simulink model "magPhase"  (R2024a)
settings: Solver=FixedStepDiscrete  StartTime=0.0  StopTime=1  RelTol=1e-3
undefined symbols (not defined in the file): dx, dy
libraries: visionsinks x4, visionsources x1
Description:
  | Sobel Edge Detection Using the MATLAB(R) Function Block
  | This example shows how to use HDL Coder(TM) to check,
  | generate, and verify HDL code for a Sobel Edge Detection
  | block built using the MATLAB Function block.
settings Model: FPTRunName=Active  Creator=The MathWorks, Inc.  LastModifiedBy=dskap
settings SolverCC: AlgebraicLoopSolver=TrustRegion
settings DataIOCC: LimitDataPoints=on  SaveFormat=Array  SignalLogging=off  ReturnWorkspaceOutputs=off
settings OptimizationCC: BlockReduction=off  ConditionallyExecuteInputs=off  DefaultParameterBehavior=Inlined  ExpressionDepthLimit=2147483647  InitFltsAndDblsToZero=on  EfficientMapNaN2IntZero=off  LifeSpan=inf
settings DebuggingCC: AlgebraicLoopMsg=error  SaveWithParameterizedLinksMsg=none  UnderspecifiedInitializationDetection=Classic  MergeDetectMultiDrivingBlocksExec=none  SignalResolutionControl=TryResolveAllWithWarning  MultiTaskDSMMsg=warning  MultiTaskCondExecSysMsg=none  SingleTaskRateTransMsg=error  IntegerOverflowMsg=none  ParameterPrecisionLossMsg=none  FcnCallInpInsideContextMsg=warning  UnconnectedInputMsg=warning  UnconnectedOutputMsg=warning  UnconnectedLineMsg=warning  AllowSymbolicDim=off  StateNameClashWarn=warning  StrictBusMsg=ErrorOnBusTreatedAsVector  SFUnexpectedBacktrackingDiag=warning  SFNoUnconditionalDefaultTransitionDiag=warning  SFExecutionAtInitializationDiag=none  IntegerSaturationMsg=none  ArithmeticOperatorsInVariantConditions=warning
settings HardwareCC: ProdBitPerPointer=32  ProdBitPerSizeT=32  ProdBitPerPtrDiffT=32  ProdLargestAtomicFloat=None  ProdIntDivRoundTo=Undefined  ProdEndianess=Unspecified  ProdWordSize=32  ProdHWDeviceType=ASIC/FPGA  TargetHWDeviceType=32-bit Generic  ProdEqTarget=off
settings ModelReferenceCC: EnableRefExpFcnMdlSchedulingChecks=on  PropagateSignalLabelsOutOfModel=off
settings SFSimCC: SimUseLocalCustomCode=off  CustomCodeUndefinedFunction=UseInterfaceOnly
settings RTWCC: RTWUseLocalCustomCode=off  GPUComputeCapability=3.5  DLArmComputeVersion=19.05
settings CodeAppCC: StateflowObjectComments=on
settings GRTTargetCC: TargetFcnLib=ansi_tfl_tmw.mat  TargetLangStandard=C89/C90 (ANSI)  CombineOutputUpdateFcns=off  GRTInterface=on
settings ConfigComp: CovMetricSettings=dw  CovSaveCumulativeToWorkspaceVar=on  CovSaveSingleToWorkspaceVar=on  CovExternalEMLEnable=off

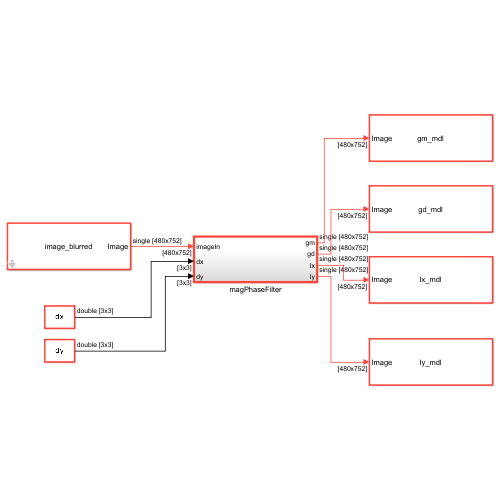
[thumbnail: Simulink's stored preview of the top-level diagram]
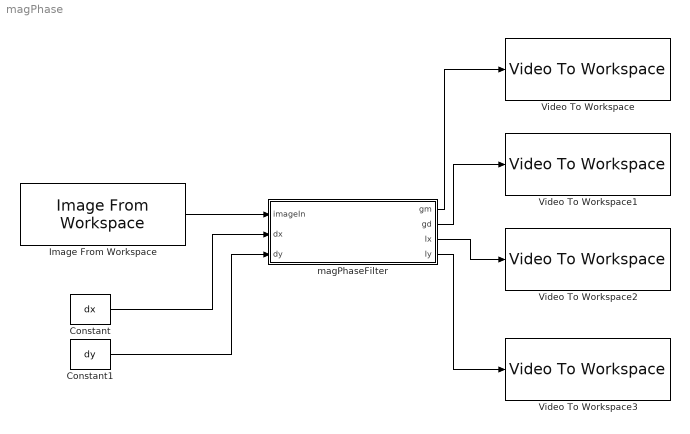
== system magPhase ==
  Constant : Constant  Value=dx  SampleTime=-1
  Constant1 : Constant  Value=dy  SampleTime=-1
  Image From Workspace : visionsources/Image From Workspace  Tag=vipblks_nd  ImageValue=image_blurred  Ts=1  imagePorts=One multidimensional signal  OutPortLabels=R|G|B  ImageDataType=Inherit from 'Value'  Signed=on  WordLength=16  sdImageDataType=sfix(16)  FractionLengthMode=User-defined  FractionLength=15
  Video To Workspace : visionsinks/Video To Workspace  VariableName=gm_mdl  NumInputs=1  DataLimit=1  DecimationFactor=1  LogFi=off  InPortLabels=R|G|B
  Video To Workspace1 : visionsinks/Video To Workspace  VariableName=gd_mdl  NumInputs=1  DataLimit=1  DecimationFactor=1  LogFi=off  InPortLabels=R|G|B
  Video To Workspace2 : visionsinks/Video To Workspace  VariableName=Ix_mdl  NumInputs=1  DataLimit=1  DecimationFactor=1  LogFi=off  InPortLabels=R|G|B
  Video To Workspace3 : visionsinks/Video To Workspace  VariableName=Iy_mdl  NumInputs=1  DataLimit=1  DecimationFactor=1  LogFi=off  InPortLabels=R|G|B
  magPhaseFilter : Subsystem  TreatAsAtomicUnit=on
  wires:
  Image From Workspace/1 -> magPhaseFilter/1(imageIn)
  magPhaseFilter/1(gm) -> Video To Workspace/1
  magPhaseFilter/2(gd) -> Video To Workspace1/1
  Constant/1 -> magPhaseFilter/2(dx)
  Constant1/1 -> magPhaseFilter/3(dy)
  magPhaseFilter/3(Ix) -> Video To Workspace2/1
  magPhaseFilter/4(Iy) -> Video To Workspace3/1

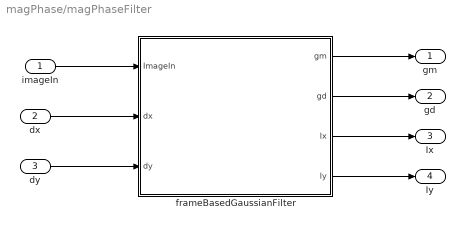
== system magPhase/magPhaseFilter ==
  imageIn : Inport
  dx : Inport  Port=2
  dy : Inport  Port=3
  frameBasedGaussianFilter : MATLAB Function  TreatAsAtomicUnit=on
  gm : Outport
  gd : Outport  Port=2
  Ix : Outport  Port=3
  Iy : Outport  Port=4
  wires:
  imageIn/1 -> frameBasedGaussianFilter/1(ImageIn)
  frameBasedGaussianFilter/1(gm) -> gm/1
  dx/1 -> frameBasedGaussianFilter/2(dx)
  dy/1 -> frameBasedGaussianFilter/3(dy)
  frameBasedGaussianFilter/2(gd) -> gd/1
  frameBasedGaussianFilter/3(Ix) -> Ix/1
  frameBasedGaussianFilter/4(Iy) -> Iy/1

== matlab function magPhase/magPhaseFilter/frameBasedGaussianFilter ==
  data: gm output; ImageIn input; dx input; dy input; gd output; Ix output; Iy output
function [gm,gd,Ix,Iy]  = frameBasedGaussianFilter(ImageIn, dx, dy)
    [gm,gd,Ix,Iy] = hdl.npufun(@gaussianKernel, [3 3], ImageIn,'NonSampleInput',dx,'NonSampleInput',dy); 
end
 
function [gm,gd,Ix,Iy] = gaussianKernel(in,dx,dy)
    %u = fi(in,1,32,15);
    
    dxTemp = in.*dx;
    Ix = sum(sum(dxTemp));

    dyTemp = in.*dy;
    Iy = sum(sum(dyTemp));

    gm = Ix.^2 + Iy.^2;   %Magnitude
    gd = atan2(Iy,Ix);    %Direction
end
